simulink library "INT_RmtAPP_DD1"  (R2016b)
settings: Solver=VariableStepAuto  StartTime=0.0  StopTime=10.0  RelTol=1e-3
settings Model: Creator=bianxuyin  LastModifiedBy=bianxuyin

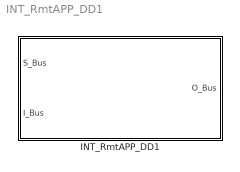
== system INT_RmtAPP_DD1 ==
  INT_RmtAPP_DD1 : Subsystem

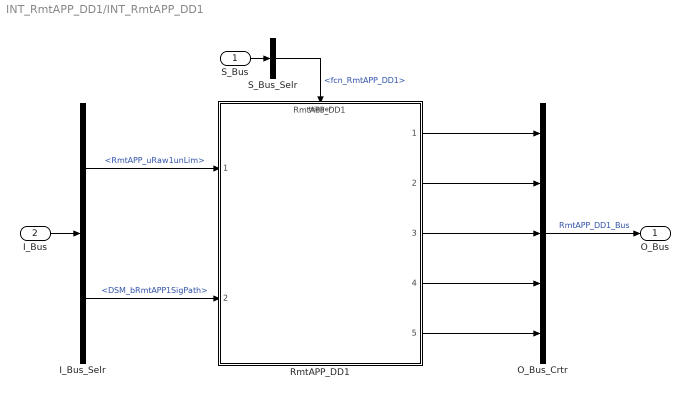
== system INT_RmtAPP_DD1/INT_RmtAPP_DD1 ==
  S_Bus : Inport
  I_Bus : Inport  Port=2
  I_Bus_Selr : BusSelector  OutputSignals=RmtAPP_uRaw1unLim,DSM_bRmtAPP1SigPath
  O_Bus_Crtr : BusCreator  Inputs=5
  RmtAPP_DD1 : ModelReference  ModelNameDialog=RmtAPP_DD1  SimulationMode=Normal  ModelReferenceVersion=1.7  TriggerPortName=function  TriggerPortTriggerType=function-call  TriggerPortStatesWhenEnabling=held
  S_Bus_Selr : BusSelector  OutputSignals=fcn_RmtAPP_DD1
  O_Bus : Outport
  wires:
  S_Bus_Selr/1 -> RmtAPP_DD1/Trigger  "<fcn_RmtAPP_DD1>"
  S_Bus/1 -> S_Bus_Selr/1
  I_Bus/1 -> I_Bus_Selr/1
  I_Bus_Selr/1 -> RmtAPP_DD1/1  "<RmtAPP_uRaw1unLim>"
  I_Bus_Selr/2 -> RmtAPP_DD1/2  "<DSM_bRmtAPP1SigPath>"
  O_Bus_Crtr/1 -> O_Bus/1  "RmtAPP_DD1_Bus"
  RmtAPP_DD1/1 -> O_Bus_Crtr/1
  RmtAPP_DD1/2 -> O_Bus_Crtr/2
  RmtAPP_DD1/3 -> O_Bus_Crtr/3
  RmtAPP_DD1/4 -> O_Bus_Crtr/4
  RmtAPP_DD1/5 -> O_Bus_Crtr/5
